simulink model "SimulinkModelEs2"  (R2023a)
settings: Solver=VariableStepAuto  StartTime=0.0  StopTime=10.0  RelTol=1e-3
libraries: vrlib x1
settings Model: Creator=pisy1  LastModifiedBy=pisy1

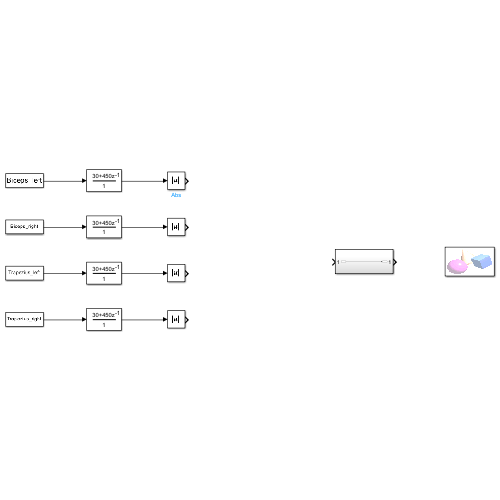
[thumbnail: Simulink's stored preview of the top-level diagram]
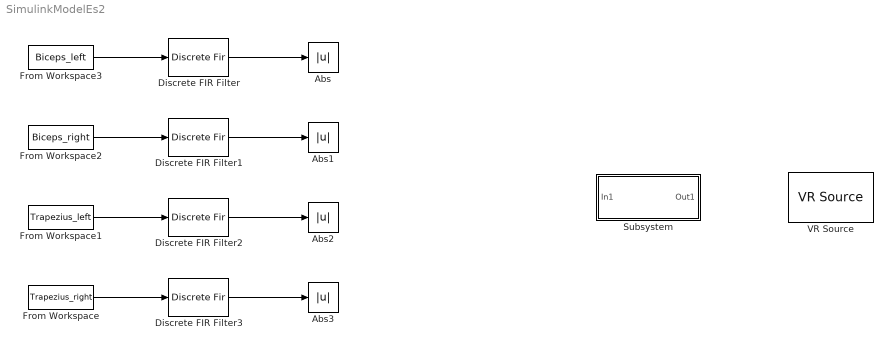
== system SimulinkModelEs2 ==
  Abs{,1..3} (4 alike) : Abs  SaturateOnIntegerOverflow=off
  Discrete FIR Filter{,1..3} (4 alike) : DiscreteFir  Coefficients=[30 450]
  From Workspace : FromWorkspace  VariableName=Trapezius_right
  From Workspace1 : FromWorkspace  VariableName=Trapezius_left
  From Workspace2 : FromWorkspace  VariableName=Biceps_right
  From Workspace3 : FromWorkspace  VariableName=Biceps_left
  Subsystem : Subsystem
  VR Source : vrlib/VR Source  InstantiateOnLoad=on  SampleTime=0.1  ViewEnable=on  RemoteChange=off  RemoteView=off  WorldFileName=8_palline_color.wrl  AutoView=off  VideoDimensions=[]  AllowVariableSize=off  FigureProperties=[]
  wires:
  From Workspace3/1 -> Discrete FIR Filter/1
  From Workspace2/1 -> Discrete FIR Filter1/1
  From Workspace1/1 -> Discrete FIR Filter2/1
  From Workspace/1 -> Discrete FIR Filter3/1
  Discrete FIR Filter/1 -> Abs/1
  Discrete FIR Filter1/1 -> Abs1/1
  Discrete FIR Filter2/1 -> Abs2/1
  Discrete FIR Filter3/1 -> Abs3/1

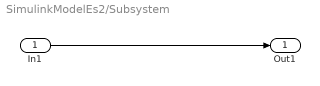
== system SimulinkModelEs2/Subsystem ==
  In1 : Inport
  Out1 : Outport
  wires:
  In1/1 -> Out1/1
